simulink model "lu4_4a"  (Simulink 7.1)
settings: Solver=ode45  StartTime=0.0  StopTime=10.0  RelTol=1e-3
libraries: simulink_extras x1
settings Model: Creator=Slavi  LastModifiedBy=Slavi

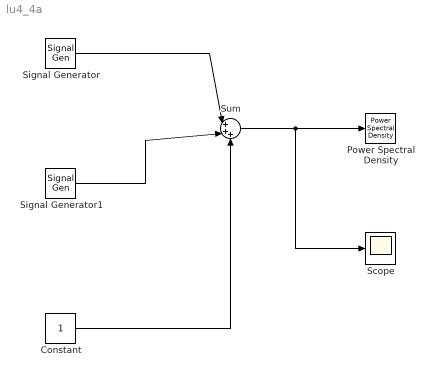
== system lu4_4a ==
  Constant : Constant  OutDataType=sfix(16)  OutScaling=2^0
  Power Spectral Density : simulink_extras/Additional Sinks/Power Spectral Density  SystemSampleTime=-1  npts=128  fftpts=512  HowOften=64  sampleT=0.1
  Scope : Scope
  Signal Generator : SignalGenerator  Amplitude=220  Frequency=50
  Signal Generator1 : SignalGenerator  WaveForm=random  Amplitude=220  Frequency=50
  Sum : Sum  Inputs=|+++  OutDataType=sfix(16)  OutScaling=2^0
  wires:
  Sum/1 -> Power Spectral Density/1, Scope/1
  Signal Generator/1 -> Sum/1
  Signal Generator1/1 -> Sum/2
  Constant/1 -> Sum/3
